simulink model "Expt2_19EE30012_Ananta_QuesB"  (R2020b)
settings: Solver=VariableStepAuto  StartTime=0.0  StopTime=0.1  RelTol=1e-3
libraries: powerlib x11, eeGeneralControl x1
settings Model: Creator=win10  LastModifiedBy=win10

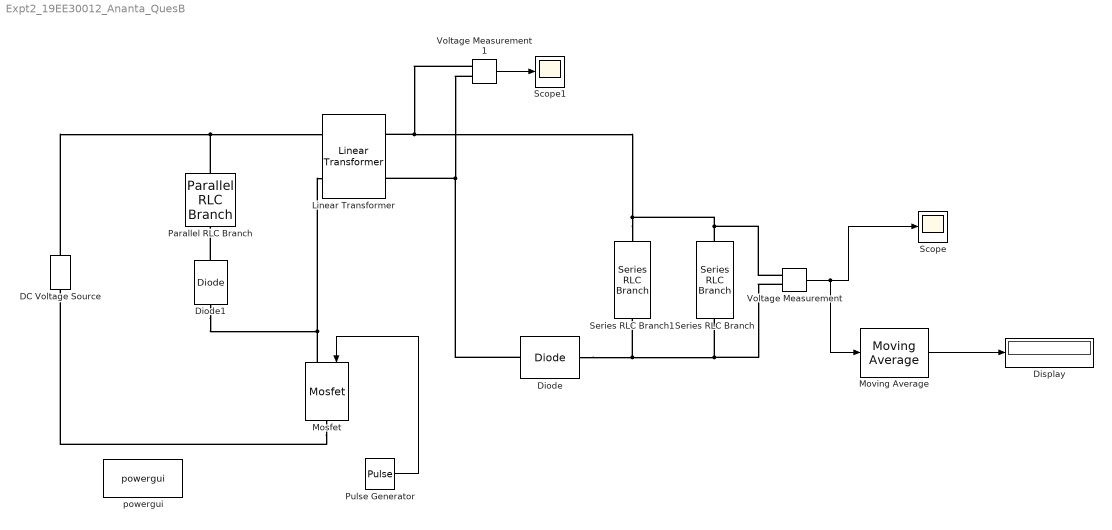
== system Expt2_19EE30012_Ananta_QuesB ==
  DC Voltage Source : powerlib/Electrical Sources/DC Voltage Source  Amplitude=24  Measurements=None
  Diode : powerlib/Power Electronics/Diode  Ron=1e-6  Lon=0  Vf=0  IC=0  UseSnubber=0  Rs=500  Cs=250e-9  Measurements=off
  Diode1 : powerlib/Power Electronics/Diode  Ron=1e-6  Lon=0  Vf=0  IC=0  UseSnubber=0  Rs=500  Cs=250e-9  Measurements=off
  Display : Display
  Linear Transformer : powerlib/Elements/Linear Transformer  UNITS=pu  NominalPower=[ 100 50]  winding1="[ 20  0 0 ]"  winding2="[ 8  0 20e-9 ]"  ThreeWindings=off  winding3=[ 315e3 0.002 0.08 ]  RmLm=[ 0 20e-6 ]  Measurements=None  DataType=off
  Mosfet : powerlib/Power Electronics/Mosfet  Ron=1e-6  Lon=0  Rd=0.01  Vfd=0  IC=0  Rs=1e5  Cs=inf  Measurements=off
  Moving Average : eeGeneralControl/Moving Average  VariantControl=Variant1  LabelModeActiveChoice=Continuous  f=60  x0=0  Ts=0
      settings: SourceProductBaseCode=PS
  Parallel RLC Branch : powerlib/Elements/Parallel RLC Branch  LConnTagsString=a  RConnTagsString=__new0  BranchType=RC  Resistance=5e3  Inductance=1e-3  SetiL0=off  InitialCurrent=0  Capacitance=50e-9  Setx0=off  InitialVoltage=0  Measurements=None
  Pulse Generator : DiscretePulseGenerator  PulseType=Time based  Period=1e-5  PulseWidth=40
  Scope : Scope
  Scope1 : Scope
  Series RLC Branch : powerlib/Elements/Series RLC Branch  LConnTagsString=__new0  RConnTagsString=__new0  BranchType=R  Resistance=1  Inductance=1e-3  SetiL0=off  InitialCurrent=0  Capacitance=1e-6  Setx0=off  InitialVoltage=0  Measurements=None
  Series RLC Branch1 : powerlib/Elements/Series RLC Branch  LConnTagsString=__new0  RConnTagsString=__new0  BranchType=C  Resistance=1  Inductance=1e-3  SetiL0=off  InitialCurrent=0  Capacitance=100e-6  Setx0=off  InitialVoltage=0  Measurements=None
  Voltage Measurement : powerlib/Measurements/Voltage Measurement  PhasorSimulation=off  OutputType=Complex  PSBequivalent=0
  Voltage Measurement1 : powerlib/Measurements/Voltage Measurement  PhasorSimulation=off  OutputType=Complex  PSBequivalent=0
  powergui : powerlib/powergui  Priority=1  SimulationMode=Discrete  SampleTime=1e-7  frequency=60  Iterations=50  frequencyindice=0  Pbase=100e6  ErrMax=1e-4  UnitsV=kV  UnitsW=MW  buscounter=0  FunctionMessages=off  echomessages=off  EnableUseOfTLC=off  CurrentSourceSwitches=off  DisableSnubberDevices=off  DisableRonSwitches=off  DisableVfSwitches=off  DisplayEquations=off  AutomaticDiscreteSolvers=off  SolverType=Tustin/Backward Euler (TBE)  Interpol=off  ExternalGateDelay=off  methode=off  Ts=100  x0status=blocks  SPID=on  SwTol=0  HookPort=off  NonlinearTolerance=1e-4  nMaxIteration=100  ContinueOnMaxIteration=off  RestoreLinks=warning  ResistiveCurrentMeasurement=off  Frange=[0:2:500]  Ylog=off  Xlog=on  ShowGrid=off  save=off  variable=ZData  structure=0  ZoomFFT=off  StartTime=0.0  cycles=1  DisplayStyle=1  fundamental=60  FreqAxis=off  MaxFrequency=1000  frequencyindicesteady=1  RmsSteady=1  display=off
  wires:
  Pulse Generator/1 -> Mosfet/1
  Moving Average/1 -> Display/1
  Voltage Measurement/1 -> Moving Average/1, Scope/1
  Voltage Measurement1/1 -> Scope1/1
  connections:
  Series RLC Branch1/LConn1 -- Diode/RConn1 -- Voltage Measurement/LConn2 -- Series RLC Branch/LConn1
  Series RLC Branch1/RConn1 -- Linear Transformer/RConn1 -- Voltage Measurement1/LConn1 -- Series RLC Branch/RConn1 -- Voltage Measurement/LConn1
  Linear Transformer/RConn2 -- Voltage Measurement1/LConn2 -- Diode/LConn1
  Mosfet/LConn1 -- Diode1/LConn1 -- Linear Transformer/LConn2
  Mosfet/RConn1 -- DC Voltage Source/LConn1
  DC Voltage Source/RConn1 -- Parallel RLC Branch/LConn1 -- Linear Transformer/LConn1
  Diode1/RConn1 -- Parallel RLC Branch/RConn1
